simulink model "parallel_8_phase_voltages"  (R2022a)
settings: Solver=FixedStepDiscrete  StartTime=0.0  StopTime=10.0  RelTol=1e-3
undefined symbols (not defined in the file or in its folder): f_c, u_dc
libraries: hdlsllib x4, simulink x2
settings Model: DataTypeOverride=Off  Creator=Andre Merx  LastModifiedBy=Andre Merx
settings SolverCC: AlgebraicLoopSolver=TrustRegion
settings DataIOCC: LimitDataPoints=on  SaveOutput=off  SaveTime=off
settings OptimizationCC: BlockReduction=off  ConditionallyExecuteInputs=off  DefaultParameterBehavior=Inlined  LifeSpan=inf
settings DebuggingCC: AlgebraicLoopMsg=error  SingleTaskRateTransMsg=error  UnconnectedInputMsg=warning  UnconnectedOutputMsg=warning  UnconnectedLineMsg=warning  AllowSymbolicDim=off  StrictBusMsg=ErrorOnBusTreatedAsVector  SFUnexpectedBacktrackingDiag=warning  SFNoUnconditionalDefaultTransitionDiag=warning  SFExecutionAtInitializationDiag=none  SFMachineParentedDataDiag=warning  ArithmeticOperatorsInVariantConditions=warning
settings HardwareCC: ProdBitPerPointer=32  ProdBitPerSizeT=32  ProdBitPerPtrDiffT=32  ProdLargestAtomicFloat=None  ProdIntDivRoundTo=Undefined  ProdEndianess=Unspecified  ProdWordSize=32  ProdHWDeviceType=ASIC/FPGA->ASIC/FPGA  ProdEqTarget=off
settings SFSimCC: SimUseLocalCustomCode=off  CustomCodeUndefinedFunction=UseInterfaceOnly
settings RTWCC: RTWUseLocalCustomCode=off
settings CodeAppCC: StateflowObjectComments=on
settings GRTTargetCC: TargetLangStandard=C89/C90 (ANSI)
settings ConfigComp: CovScope=ReferencedModels  CovMetricSettings=dw  CovSaveCumulativeToWorkspaceVar=on  CovSaveSingleToWorkspaceVar=on  CovExternalEMLEnable=off  CovSFcnEnable=off

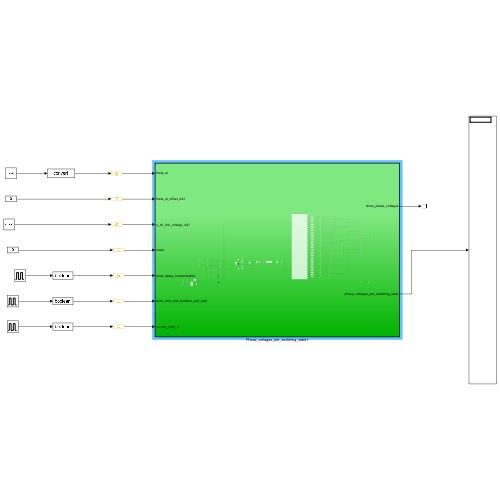
[thumbnail: Simulink's stored preview of the top-level diagram]
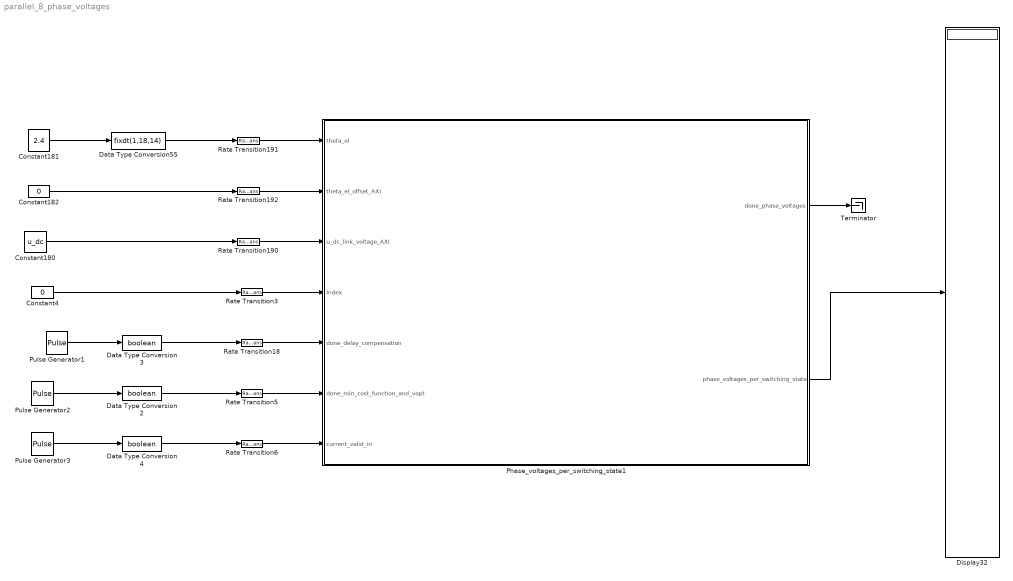
== system parallel_8_phase_voltages ==
  Constant180 : Constant  Value=u_dc  OutDataTypeStr=single  SampleTime=-1
  Constant181 : Constant  Value=2.4
  Constant182 : Constant  Value=0  OutDataTypeStr=fixdt(1,18,14)  SampleTime=-1
  Constant4 : Constant  Value=0  OutDataTypeStr=int32  SampleTime=-1
  Data Type Conversion2 : DataTypeConversion  OutDataTypeStr=boolean  SaturateOnIntegerOverflow=off  RndMeth=Floor
  Data Type Conversion3 : DataTypeConversion  OutDataTypeStr=boolean  SaturateOnIntegerOverflow=off  RndMeth=Floor
  Data Type Conversion4 : DataTypeConversion  OutDataTypeStr=boolean  SaturateOnIntegerOverflow=off  RndMeth=Floor
  Data Type Conversion55 : DataTypeConversion  OutDataTypeStr=fixdt(1,18,14)  SaturateOnIntegerOverflow=off  RndMeth=Floor
  Display32 : Display
  Phase_voltages_per_switching_state1 : Subsystem  TreatAsAtomicUnit=on
  Pulse Generator1 : DiscretePulseGenerator  PulseType=Time based  Period=1/f_c
  Pulse Generator2 : DiscretePulseGenerator  PulseType=Time based  Period=1/f_c
  Pulse Generator3 : DiscretePulseGenerator  PulseType=Time based  Period=1/f_c
  Rate Transition{3,5..6,18,190..192} (7 alike) : RateTransition  OutPortSampleTime=Rt
  Terminator : Terminator
  wires:
  Constant181/1 -> Data Type Conversion55/1
  Data Type Conversion55/1 -> Rate Transition191/1
  Constant180/1 -> Rate Transition190/1
  Constant182/1 -> Rate Transition192/1
  Rate Transition192/1 -> Phase_voltages_per_switching_state1/2(theta_el_offset_AXI)
  Phase_voltages_per_switching_state1/2(phase_voltages_per_switching_state) -> Display32/1
  Rate Transition191/1 -> Phase_voltages_per_switching_state1/1(theta_el)
  Rate Transition190/1 -> Phase_voltages_per_switching_state1/3(u_dc_link_voltage_AXI)
  Phase_voltages_per_switching_state1/1(done_phase_voltages) -> Terminator/1
  Pulse Generator2/1 -> Data Type Conversion2/1
  Rate Transition5/1 -> Phase_voltages_per_switching_state1/6(done_min_cost_function_and_vopt)
  Pulse Generator1/1 -> Data Type Conversion3/1
  Pulse Generator3/1 -> Data Type Conversion4/1
  Constant4/1 -> Rate Transition3/1
  Data Type Conversion4/1 -> Rate Transition6/1
  Data Type Conversion3/1 -> Rate Transition18/1
  Rate Transition18/1 -> Phase_voltages_per_switching_state1/5(done_delay_compensation)
  Rate Transition6/1 -> Phase_voltages_per_switching_state1/7(current_valid_in)
  Data Type Conversion2/1 -> Rate Transition5/1
  Rate Transition3/1 -> Phase_voltages_per_switching_state1/4(Index)

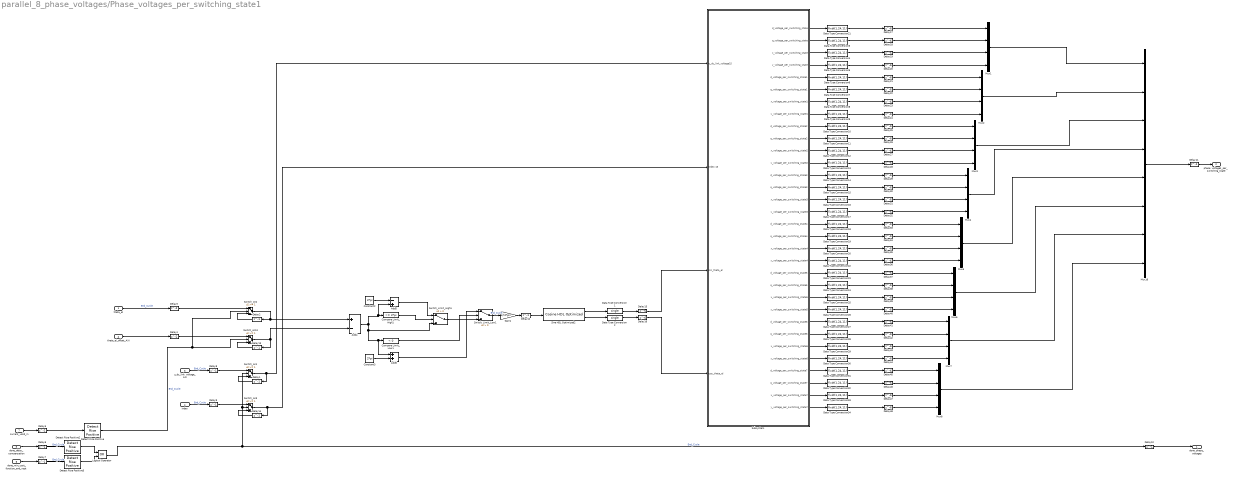
== system parallel_8_phase_voltages/Phase_voltages_per_switching_state1 ==
  theta_el : Inport
  theta_el_offset_AXI : Inport  Port=2
  u_dc_link_voltage_AXI : Inport  Port=3
  Index : Inport  Port=4
  done_delay_compensation : Inport  Port=5
  done_min_cost_function_and_vopt : Inport  Port=6
  current_valid_in : Inport  Port=7
  Add4 : Sum  Inputs=+-  OutDataTypeStr=Inherit: Same as first input
  Add5 : Sum  Inputs=-+  OutDataTypeStr=Inherit: Same as first input
  Add6 : Sum  OutDataTypeStr=Inherit: Same as first input
  Compare Limit_High1 : simulink/Logic and Bit Operations/Compare To Constant  relop=>=  const=2*pi  OutDataTypeStr=boolean
  Compare Limit_Low1 : simulink/Logic and Bit Operations/Compare To Constant  relop=<  const=0  OutDataTypeStr=boolean
  Constant2 : Constant  Value=2*pi  OutDataTypeStr=fixdt(1,18,14)  SampleTime=1/100000000
  Constant3 : Constant  Value=2*pi  OutDataTypeStr=fixdt(1,18,14)  SampleTime=1/100000000
  Data Type Conversion1 : DataTypeConversion  OutDataTypeStr=single  SaturateOnIntegerOverflow=off  RndMeth=Floor
  Data Type Conversion{3..34} (32 alike) : DataTypeConversion  OutDataTypeStr=fixdt(1,24,11)  SaturateOnIntegerOverflow=off  RndMeth=Floor
  Data Type Conversion2 : DataTypeConversion  OutDataTypeStr=single  SaturateOnIntegerOverflow=off  RndMeth=Floor
  Delay{1..2,6..14} (11 alike) : Delay  DelayLength=1
  Delay{15..48} (34 alike) : Delay  DelayLength=6
  Delay3 : Delay
  Delay4 : Delay
  Delay5 : Delay
  Detect Rise Positive : hdlsllib/Logic and Bit Operations/Detect Rise Positive  vinit=0  OutDataTypeStr=boolean
      settings: SourceProductBaseCode=SL
  Detect Rise Positive2 : hdlsllib/Logic and Bit Operations/Detect Rise Positive  vinit=0  OutDataTypeStr=boolean
      settings: SourceProductBaseCode=SL
  Detect Rise Positive3 : hdlsllib/Logic and Bit Operations/Detect Rise Positive  vinit=0  OutDataTypeStr=boolean
      settings: SourceProductBaseCode=SL
  Gain1 : Gain  Gain=1/(2*pi)  OutDataTypeStr=Inherit: Same as input  ParamDataTypeStr=Inherit: Same as input
  Logical Operator : Logic  Operator=OR  AllPortsSameDT=off  OutDataTypeStr=boolean
  Mux{1..8} (8 alike) : Mux
  Mux16 : Mux  Inputs=8
  Sine HDL Optimized2 : hdlsllib/Lookup Tables/Cosine HDL Optimized  OutputFormula=sin(2*pi*u) and cos(2*pi*u)  NumDataPoints=512  TableDataTypeStr=fixdt(1,15,14)  SimulateLUTROMDelay=off
      settings: SourceProductBaseCode=SL
  Subsystem : Subsystem
  Switch_Limit_High1 : Switch  Criteria=u2 > Threshold  SaturateOnIntegerOverflow=off  InputSameDT=off  OutDataTypeStr=Inherit: Same as first input
  Switch_Limit_Low1 : Switch  Criteria=u2 > Threshold  SaturateOnIntegerOverflow=off  InputSameDT=off  OutDataTypeStr=Inherit: Same as first input
  Switch_on1 : Switch  Threshold=1  OutDataTypeStr=single  RndMeth=Simplest  SaturateOnIntegerOverflow=off  InputSameDT=off
  Switch_on13 : Switch  Threshold=1  RndMeth=Simplest  SaturateOnIntegerOverflow=off  InputSameDT=off  OutDataTypeStr=Inherit: Same as first input
  Switch_on2 : Switch  Threshold=1  RndMeth=Simplest  SaturateOnIntegerOverflow=off  InputSameDT=off  OutDataTypeStr=Inherit: Same as first input
  Switch_on3 : Switch  Threshold=1  OutDataTypeStr=int32  RndMeth=Simplest  SaturateOnIntegerOverflow=off  InputSameDT=off
  done_phase_voltages : Outport
  phase_voltages_per_switching_state : Outport  Port=2
  wires:
  Delay14/1 -> Switch_on3/3
  Delay13/1 -> Switch_on13/3
  Switch_on13/1 -> Delay13/1, Add4/2
  u_dc_link_voltage_AXI/1 -> Delay8/1  "End_Cycle"
  Switch_on1/1 -> Subsystem/1(u_dc_link_voltage15), Delay1/1
  Logical Operator/1 -> Delay10/1, Switch_on3/2, Switch_on1/2  "End_Cycle"
  Delay1/1 -> Switch_on1/3
  Index/1 -> Delay9/1  "End_Cycle"
  Switch_on3/1 -> Delay14/1, Subsystem/2(Index 15)
  Mux1/1 -> Mux16/1
  Mux2/1 -> Mux16/2
  Mux3/1 -> Mux16/3
  Mux4/1 -> Mux16/4
  Mux5/1 -> Mux16/5
  Mux6/1 -> Mux16/6
  Mux7/1 -> Mux16/7
  Mux8/1 -> Mux16/8
  Mux16/1 -> Delay11/1
  current_valid_in/1 -> Delay5/1
  done_delay_compensation/1 -> Delay6/1
  done_min_cost_function_and_vopt/1 -> Delay7/1
  theta_el/1 -> Delay3/1  "End_Cycle"
  Add4/1 -> Switch_Limit_High1/3, Add6/1, Compare Limit_Low1/1, Add5/2, Compare Limit_High1/1
  Compare Limit_Low1/1 -> Switch_Limit_Low1/2
  Add5/1 -> Switch_Limit_High1/1
  theta_el_offset_AXI/1 -> Delay4/1
  Constant3/1 -> Add6/2
  Constant2/1 -> Add5/1
  Compare Limit_High1/1 -> Switch_Limit_High1/2
  Add6/1 -> Switch_Limit_Low1/1
  Switch_Limit_High1/1 -> Switch_Limit_Low1/3
  Delay2/1 -> Switch_on2/3
  Switch_on2/1 -> Add4/1, Delay2/1
  Detect Rise Positive/1 -> Switch_on2/2, Switch_on13/2  "End_Cycle"
  Delay3/1 -> Switch_on2/1
  Delay4/1 -> Switch_on13/1
  Delay5/1 -> Detect Rise Positive/1
  Delay6/1 -> Detect Rise Positive2/1
  Delay7/1 -> Detect Rise Positive3/1
  Delay8/1 -> Switch_on1/1
  Delay9/1 -> Switch_on3/1
  Delay10/1 -> done_phase_voltages/1
  Delay11/1 -> phase_voltages_per_switching_state/1
  Sine HDL Optimized2/2 -> Data Type Conversion2/1
  Subsystem/1(d_voltage_per_switching_state) -> Data Type Conversion21/1
  Subsystem/2(q_voltage_per_switching_state) -> Data Type Conversion3/1
  Subsystem/3(x_voltage_per_switching_state) -> Data Type Conversion4/1
  Subsystem/4(y_voltage_per_switching_state) -> Data Type Conversion5/1
  Subsystem/5(d_voltage_per_switching_state1) -> Data Type Conversion6/1
  Subsystem/6(q_voltage_per_switching_state1) -> Data Type Conversion7/1
  Subsystem/7(x_voltage_per_switching_state1) -> Data Type Conversion8/1
  Subsystem/8(y_voltage_per_switching_state1) -> Data Type Conversion9/1
  Subsystem/9(d_voltage_per_switching_state2) -> Data Type Conversion10/1
  Subsystem/10(q_voltage_per_switching_state2) -> Data Type Conversion11/1
  Subsystem/11(x_voltage_per_switching_state2) -> Data Type Conversion12/1
  Subsystem/12(y_voltage_per_switching_state2) -> Data Type Conversion13/1
  Subsystem/13(d_voltage_per_switching_state3) -> Data Type Conversion14/1
  Subsystem/14(q_voltage_per_switching_state3) -> Data Type Conversion15/1
  Subsystem/15(x_voltage_per_switching_state3) -> Data Type Conversion16/1
  Subsystem/16(y_voltage_per_switching_state3) -> Data Type Conversion17/1
  Subsystem/17(d_voltage_per_switching_state4) -> Data Type Conversion18/1
  Subsystem/18(q_voltage_per_switching_state4) -> Data Type Conversion19/1
  Subsystem/19(x_voltage_per_switching_state4) -> Data Type Conversion20/1
  Subsystem/20(y_voltage_per_switching_state4) -> Data Type Conversion22/1
  Subsystem/21(d_voltage_per_switching_state5) -> Data Type Conversion23/1
  Subsystem/22(q_voltage_per_switching_state5) -> Data Type Conversion24/1
  Subsystem/23(x_voltage_per_switching_state5) -> Data Type Conversion25/1
  Subsystem/24(y_voltage_per_switching_state5) -> Data Type Conversion26/1
  Subsystem/25(d_voltage_per_switching_state6) -> Data Type Conversion27/1
  Subsystem/26(q_voltage_per_switching_state6) -> Data Type Conversion28/1
  Subsystem/27(x_voltage_per_switching_state6) -> Data Type Conversion29/1
  Subsystem/28(y_voltage_per_switching_state6) -> Data Type Conversion30/1
  Subsystem/29(d_voltage_per_switching_state7) -> Data Type Conversion31/1
  Subsystem/30(q_voltage_per_switching_state7) -> Data Type Conversion32/1
  Subsystem/31(x_voltage_per_switching_state7) -> Data Type Conversion33/1
  Subsystem/32(y_voltage_per_switching_state7) -> Data Type Conversion34/1
  Sine HDL Optimized2/1 -> Data Type Conversion1/1
  Data Type Conversion2/1 -> Delay16/1
  Data Type Conversion1/1 -> Delay15/1
  Gain1/1 -> Delay12/1
  Delay12/1 -> Sine HDL Optimized2/1
  Switch_Limit_Low1/1 -> Gain1/1  "End_Cycle"
  Data Type Conversion21/1 -> Delay17/1
  Data Type Conversion3/1 -> Delay18/1
  Data Type Conversion4/1 -> Delay19/1
  Data Type Conversion5/1 -> Delay20/1
  Data Type Conversion6/1 -> Delay21/1
  Data Type Conversion7/1 -> Delay22/1
  Data Type Conversion8/1 -> Delay23/1
  Data Type Conversion9/1 -> Delay24/1
  Data Type Conversion10/1 -> Delay25/1
  Data Type Conversion11/1 -> Delay26/1
  Data Type Conversion12/1 -> Delay27/1
  Data Type Conversion13/1 -> Delay28/1
  Data Type Conversion14/1 -> Delay29/1
  Data Type Conversion15/1 -> Delay30/1
  Data Type Conversion16/1 -> Delay31/1
  Data Type Conversion17/1 -> Delay32/1
  Data Type Conversion18/1 -> Delay33/1
  Data Type Conversion19/1 -> Delay34/1
  Data Type Conversion20/1 -> Delay35/1
  Data Type Conversion22/1 -> Delay36/1
  Data Type Conversion23/1 -> Delay37/1
  Data Type Conversion24/1 -> Delay38/1
  Data Type Conversion25/1 -> Delay39/1
  Data Type Conversion26/1 -> Delay40/1
  Data Type Conversion27/1 -> Delay41/1
  Data Type Conversion28/1 -> Delay42/1
  Data Type Conversion29/1 -> Delay43/1
  Data Type Conversion30/1 -> Delay44/1
  Data Type Conversion31/1 -> Delay45/1
  Data Type Conversion32/1 -> Delay46/1
  Data Type Conversion33/1 -> Delay47/1
  Data Type Conversion34/1 -> Delay48/1
  Delay15/1 -> Subsystem/3(sin_theta_el)
  Delay16/1 -> Subsystem/4(cos_theta_el)
  Delay17/1 -> Mux1/1
  Delay18/1 -> Mux1/2
  Delay19/1 -> Mux1/3
  Delay20/1 -> Mux1/4
  Delay21/1 -> Mux2/1
  Delay22/1 -> Mux2/2
  Delay23/1 -> Mux2/3
  Delay24/1 -> Mux2/4
  Delay25/1 -> Mux3/1
  Delay26/1 -> Mux3/2
  Delay27/1 -> Mux3/3
  Delay28/1 -> Mux3/4
  Delay29/1 -> Mux4/1
  Delay30/1 -> Mux4/2
  Delay31/1 -> Mux4/3
  Delay32/1 -> Mux4/4
  Delay33/1 -> Mux5/1
  Delay34/1 -> Mux5/2
  Delay35/1 -> Mux5/3
  Delay36/1 -> Mux5/4
  Delay37/1 -> Mux6/1
  Delay38/1 -> Mux6/2
  Delay39/1 -> Mux6/3
  Delay40/1 -> Mux6/4
  Delay41/1 -> Mux7/1
  Delay42/1 -> Mux7/2
  Delay43/1 -> Mux7/3
  Delay44/1 -> Mux7/4
  Delay45/1 -> Mux8/1
  Delay46/1 -> Mux8/2
  Delay47/1 -> Mux8/3
  Delay48/1 -> Mux8/4
  Detect Rise Positive2/1 -> Logical Operator/1  "End_Cycle"
  Detect Rise Positive3/1 -> Logical Operator/2  "End_Cycle"

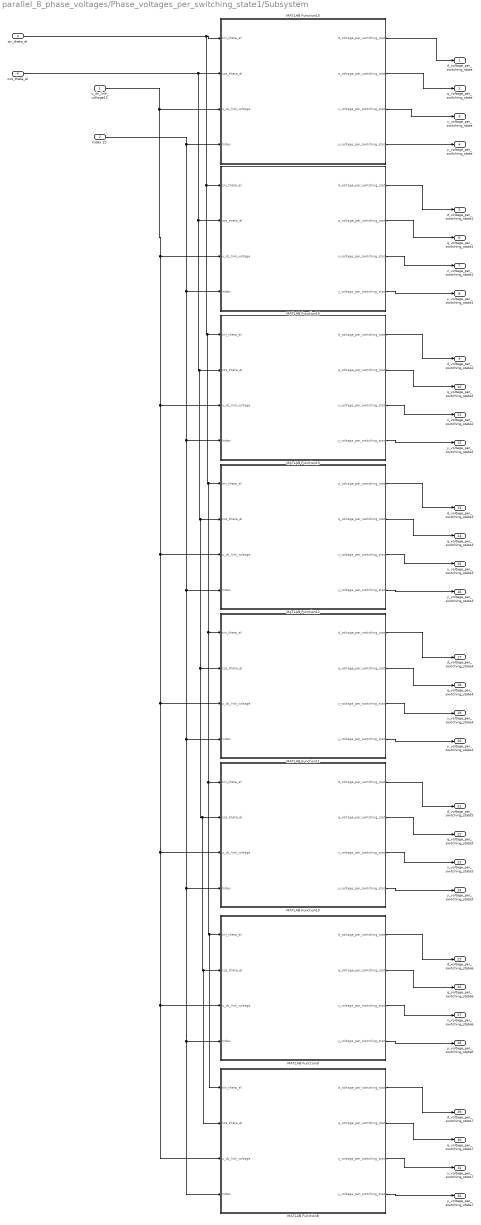
== system parallel_8_phase_voltages/Phase_voltages_per_switching_state1/Subsystem ==
  u_dc_link_voltage15 : Inport
  Index 15 : Inport  Port=2
  sin_theta_el : Inport  Port=3
  cos_theta_el : Inport  Port=4
  MATLAB Function10 : MATLAB Function  TreatAsAtomicUnit=on  SystemSampleTime=1/100000000
  MATLAB Function11 : MATLAB Function  TreatAsAtomicUnit=on  SystemSampleTime=1/100000000
  MATLAB Function12 : MATLAB Function  TreatAsAtomicUnit=on  SystemSampleTime=1/100000000
  MATLAB Function13 : MATLAB Function  TreatAsAtomicUnit=on  SystemSampleTime=1/100000000
  MATLAB Function14 : MATLAB Function  TreatAsAtomicUnit=on  SystemSampleTime=1/100000000
  MATLAB Function15 : MATLAB Function  TreatAsAtomicUnit=on  SystemSampleTime=1/100000000
  MATLAB Function8 : MATLAB Function  TreatAsAtomicUnit=on  SystemSampleTime=1/100000000
  MATLAB Function9 : MATLAB Function  TreatAsAtomicUnit=on  SystemSampleTime=1/100000000
  d_voltage_per_switching_state : Outport
  q_voltage_per_switching_state : Outport  Port=2
  x_voltage_per_switching_state : Outport  Port=3
  y_voltage_per_switching_state : Outport  Port=4
  d_voltage_per_switching_state1 : Outport  Port=5
  q_voltage_per_switching_state1 : Outport  Port=6
  x_voltage_per_switching_state1 : Outport  Port=7
  y_voltage_per_switching_state1 : Outport  Port=8
  d_voltage_per_switching_state2 : Outport  Port=9
  q_voltage_per_switching_state2 : Outport  Port=10
  x_voltage_per_switching_state2 : Outport  Port=11
  y_voltage_per_switching_state2 : Outport  Port=12
  d_voltage_per_switching_state3 : Outport  Port=13
  q_voltage_per_switching_state3 : Outport  Port=14
  x_voltage_per_switching_state3 : Outport  Port=15
  y_voltage_per_switching_state3 : Outport  Port=16
  d_voltage_per_switching_state4 : Outport  Port=17
  q_voltage_per_switching_state4 : Outport  Port=18
  x_voltage_per_switching_state4 : Outport  Port=19
  y_voltage_per_switching_state4 : Outport  Port=20
  d_voltage_per_switching_state5 : Outport  Port=21
  q_voltage_per_switching_state5 : Outport  Port=22
  x_voltage_per_switching_state5 : Outport  Port=23
  y_voltage_per_switching_state5 : Outport  Port=24
  d_voltage_per_switching_state6 : Outport  Port=25
  q_voltage_per_switching_state6 : Outport  Port=26
  x_voltage_per_switching_state6 : Outport  Port=27
  y_voltage_per_switching_state6 : Outport  Port=28
  d_voltage_per_switching_state7 : Outport  Port=29
  q_voltage_per_switching_state7 : Outport  Port=30
  x_voltage_per_switching_state7 : Outport  Port=31
  y_voltage_per_switching_state7 : Outport  Port=32
  wires:
  MATLAB Function11/4(y_voltage_per_switching_state) -> y_voltage_per_switching_state4/1
  MATLAB Function10/3(x_voltage_per_switching_state) -> x_voltage_per_switching_state5/1
  MATLAB Function8/1(d_voltage_per_switching_state) -> d_voltage_per_switching_state7/1
  MATLAB Function8/2(q_voltage_per_switching_state) -> q_voltage_per_switching_state7/1
  MATLAB Function11/1(d_voltage_per_switching_state) -> d_voltage_per_switching_state4/1
  MATLAB Function12/3(x_voltage_per_switching_state) -> x_voltage_per_switching_state3/1
  MATLAB Function15/2(q_voltage_per_switching_state) -> q_voltage_per_switching_state/1
  MATLAB Function8/3(x_voltage_per_switching_state) -> x_voltage_per_switching_state7/1
  MATLAB Function11/3(x_voltage_per_switching_state) -> x_voltage_per_switching_state4/1
  MATLAB Function10/4(y_voltage_per_switching_state) -> y_voltage_per_switching_state5/1
  MATLAB Function11/2(q_voltage_per_switching_state) -> q_voltage_per_switching_state4/1
  MATLAB Function12/1(d_voltage_per_switching_state) -> d_voltage_per_switching_state3/1
  MATLAB Function12/4(y_voltage_per_switching_state) -> y_voltage_per_switching_state3/1
  MATLAB Function13/2(q_voltage_per_switching_state) -> q_voltage_per_switching_state2/1
  MATLAB Function10/1(d_voltage_per_switching_state) -> d_voltage_per_switching_state5/1
  MATLAB Function10/2(q_voltage_per_switching_state) -> q_voltage_per_switching_state5/1
  MATLAB Function13/4(y_voltage_per_switching_state) -> y_voltage_per_switching_state2/1
  MATLAB Function8/4(y_voltage_per_switching_state) -> y_voltage_per_switching_state7/1
  MATLAB Function13/1(d_voltage_per_switching_state) -> d_voltage_per_switching_state2/1
  MATLAB Function13/3(x_voltage_per_switching_state) -> x_voltage_per_switching_state2/1
  MATLAB Function12/2(q_voltage_per_switching_state) -> q_voltage_per_switching_state3/1
  MATLAB Function15/1(d_voltage_per_switching_state) -> d_voltage_per_switching_state/1
  MATLAB Function15/4(y_voltage_per_switching_state) -> y_voltage_per_switching_state/1
  MATLAB Function15/3(x_voltage_per_switching_state) -> x_voltage_per_switching_state/1
  u_dc_link_voltage15/1 -> MATLAB Function8/3(u_dc_link_voltage), MATLAB Function9/3(u_dc_link_voltage), MATLAB Function10/3(u_dc_link_voltage), MATLAB Function11/3(u_dc_link_voltage), MATLAB Function12/3(u_dc_link_voltage), MATLAB Function13/3(u_dc_link_voltage), MATLAB Function14/3(u_dc_link_voltage), MATLAB Function15/3(u_dc_link_voltage)
  MATLAB Function14/4(y_voltage_per_switching_state) -> y_voltage_per_switching_state1/1
  MATLAB Function14/3(x_voltage_per_switching_state) -> x_voltage_per_switching_state1/1
  MATLAB Function14/1(d_voltage_per_switching_state) -> d_voltage_per_switching_state1/1
  MATLAB Function14/2(q_voltage_per_switching_state) -> q_voltage_per_switching_state1/1
  Index 15/1 -> MATLAB Function15/4(Index), MATLAB Function10/4(Index), MATLAB Function8/4(Index), MATLAB Function9/4(Index), MATLAB Function11/4(Index), MATLAB Function12/4(Index), MATLAB Function13/4(Index), MATLAB Function14/4(Index)
  MATLAB Function9/3(x_voltage_per_switching_state) -> x_voltage_per_switching_state6/1
  MATLAB Function9/2(q_voltage_per_switching_state) -> q_voltage_per_switching_state6/1
  MATLAB Function9/1(d_voltage_per_switching_state) -> d_voltage_per_switching_state6/1
  MATLAB Function9/4(y_voltage_per_switching_state) -> y_voltage_per_switching_state6/1
  sin_theta_el/1 -> MATLAB Function14/1(sin_theta_el), MATLAB Function8/1(sin_theta_el), MATLAB Function9/1(sin_theta_el), MATLAB Function10/1(sin_theta_el), MATLAB Function11/1(sin_theta_el), MATLAB Function12/1(sin_theta_el), MATLAB Function13/1(sin_theta_el), MATLAB Function15/1(sin_theta_el)
  cos_theta_el/1 -> MATLAB Function15/2(cos_theta_el), MATLAB Function8/2(cos_theta_el), MATLAB Function9/2(cos_theta_el), MATLAB Function10/2(cos_theta_el), MATLAB Function11/2(cos_theta_el), MATLAB Function12/2(cos_theta_el), MATLAB Function13/2(cos_theta_el), MATLAB Function14/2(cos_theta_el)

== matlab function parallel_8_phase_voltages/Phase_voltages_per_switching_state1/Subsystem/MATLAB Function9 ==
  data: sin_theta_el input; cos_theta_el input; d_voltage_per_switching_state output; u_dc_link_voltage input; Index input; q_voltage_per_switching_state output; x_voltage_per_switching_state output; y_voltage_per_switching_state output
function [d_voltage_per_switching_state, q_voltage_per_switching_state, x_voltage_per_switching_state, y_voltage_per_switching_state] = fcn(sin_theta_el, cos_theta_el, u_dc_link_voltage, Index)
      
        % Initial condition
            Index = Index+1;

    
        % Swichtingstates factors alpha beta x y
        Factors_alpha_beta_x_y = single([-0.288675134594813	 0.0446581987385205  -0.455341801261480	  -0.122008467928146    -0.455341801261480	-0.122008467928146	-0.622008467928146	-0.288675134594813;
                                         -0.166666666666667	-0.166666666666667	  0.122008467928146	   0.122008467928146    -0.455341801261480	-0.455341801261480	-0.166666666666667	-0.166666666666667;
                                         0.288675134594813	 0.622008467928146	  0.122008467928146	   0.455341801261480     0.122008467928146	 0.455341801261480	-0.0446581987385205  0.288675134594813;
                                         -0.166666666666667	-0.166666666666667	 -0.455341801261480	  -0.455341801261480     0.122008467928146	 0.122008467928146	-0.166666666666667	-0.166666666666667]);
        
        % Park-Transformation of the switchingstates factors
        Factors_d_q_x_y =single(zeros(4,1));
    
        Factors_d_q_x_y(3,1) = Factors_alpha_beta_x_y(3,Index);
        Factors_d_q_x_y(4,1) = Factors_alpha_beta_x_y(4,Index);
       
        Factors_d_q_x_y(1,1) = cos_theta_el*Factors_alpha_beta_x_y(1,Index)+sin_theta_el*Factors_alpha_beta_x_y(2,Index);
        Factors_d_q_x_y(2,1) = -sin_theta_el*Factors_alpha_beta_x_y(1,Index)+cos_theta_el*Factors_alpha_beta_x_y(2,Index);
    
        %Calculation of the voltages per switching state in alpha beta coordinates
        d_q_x_y_voltages_per_switching_state = single(u_dc_link_voltage*Factors_d_q_x_y);
    
        d_voltage_per_switching_state = d_q_x_y_voltages_per_switching_state(1,1);
        q_voltage_per_switching_state = d_q_x_y_voltages_per_switching_state(2,1);
        x_voltage_per_switching_state = d_q_x_y_voltages_per_switching_state(3,1);
        y_voltage_per_switching_state = d_q_x_y_voltages_per_switching_state(4,1);
    

end

== matlab function parallel_8_phase_voltages/Phase_voltages_per_switching_state1/Subsystem/MATLAB Function10 ==
  data: sin_theta_el input; cos_theta_el input; d_voltage_per_switching_state output; u_dc_link_voltage input; Index input; q_voltage_per_switching_state output; x_voltage_per_switching_state output; y_voltage_per_switching_state output
function [d_voltage_per_switching_state, q_voltage_per_switching_state, x_voltage_per_switching_state, y_voltage_per_switching_state] = fcn(sin_theta_el, cos_theta_el, u_dc_link_voltage, Index)
      
        % Initial condition
            Index = Index+1;

        % Swichtingstates factors alpha beta x y
        Factors_alpha_beta_x_y = single([0.288675134594813	 0.622008467928146	 0.122008467928146	 0.455341801261480    0.122008467928146	 0.455341801261480	-0.0446581987385205  0.288675134594813;
                                         -0.166666666666667	-0.166666666666667	 0.122008467928146	 0.122008467928146   -0.455341801261480	-0.455341801261480	-0.166666666666667	-0.166666666666667;
                                         -0.288675134594813	 0.0446581987385205	-0.455341801261480	-0.122008467928146   -0.455341801261480	-0.122008467928146	-0.622008467928146	-0.288675134594813;
                                         -0.166666666666667	-0.166666666666667	-0.455341801261480	-0.455341801261480    0.122008467928146	 0.122008467928146	-0.166666666666667	-0.166666666666667]);
        
        % Park-Transformation of the switchingstates factors
        Factors_d_q_x_y =single(zeros(4,1));
    
        Factors_d_q_x_y(3,1) = Factors_alpha_beta_x_y(3,Index);
        Factors_d_q_x_y(4,1) = Factors_alpha_beta_x_y(4,Index);
       
        Factors_d_q_x_y(1,1) = cos_theta_el*Factors_alpha_beta_x_y(1,Index)+sin_theta_el*Factors_alpha_beta_x_y(2,Index);
        Factors_d_q_x_y(2,1) = -sin_theta_el*Factors_alpha_beta_x_y(1,Index)+cos_theta_el*Factors_alpha_beta_x_y(2,Index);
    
        %Calculation of the voltages per switching state in alpha beta coordinates
        d_q_x_y_voltages_per_switching_state = single(u_dc_link_voltage*Factors_d_q_x_y);
    
        d_voltage_per_switching_state = d_q_x_y_voltages_per_switching_state(1,1);
        q_voltage_per_switching_state = d_q_x_y_voltages_per_switching_state(2,1);
        x_voltage_per_switching_state = d_q_x_y_voltages_per_switching_state(3,1);
        y_voltage_per_switching_state = d_q_x_y_voltages_per_switching_state(4,1);
    

end

== matlab function parallel_8_phase_voltages/Phase_voltages_per_switching_state1/Subsystem/MATLAB Function11 ==
  data: sin_theta_el input; cos_theta_el input; d_voltage_per_switching_state output; u_dc_link_voltage input; Index input; q_voltage_per_switching_state output; x_voltage_per_switching_state output; y_voltage_per_switching_state output
function [d_voltage_per_switching_state, q_voltage_per_switching_state, x_voltage_per_switching_state, y_voltage_per_switching_state] = fcn(sin_theta_el, cos_theta_el, u_dc_link_voltage, Index)
      
        % Initial condition
            Index = Index+1;

    
        % Swichtingstates factors alpha beta x y
        Factors_alpha_beta_x_y = single([0	                 0.333333333333333	-0.166666666666667	  0.166666666666667    -0.166666666666667	  0.166666666666667	    -0.333333333333333	 0;
                                        -0.333333333333333	-0.333333333333333	-0.0446581987385205	 -0.0446581987385205   -0.622008467928146	 -0.622008467928146	    -0.333333333333333	-0.333333333333333;
                                         0	                 0.333333333333333	-0.166666666666667	  0.166666666666667    -0.166666666666667	  0.166666666666667	    -0.333333333333333	 0;
                                        -0.333333333333333	-0.333333333333333	-0.622008467928146	 -0.622008467928146    -0.0446581987385205   -0.0446581987385205	-0.333333333333333	-0.333333333333333]);
        
        % Park-Transformation of the switchingstates factors
        Factors_d_q_x_y =single(zeros(4,1));
    
        Factors_d_q_x_y(3,1) = Factors_alpha_beta_x_y(3,Index);
        Factors_d_q_x_y(4,1) = Factors_alpha_beta_x_y(4,Index);

        Factors_d_q_x_y(1,1) = cos_theta_el*Factors_alpha_beta_x_y(1,Index)+sin_theta_el*Factors_alpha_beta_x_y(2,Index);
        Factors_d_q_x_y(2,1) = -sin_theta_el*Factors_alpha_beta_x_y(1,Index)+cos_theta_el*Factors_alpha_beta_x_y(2,Index);
    
        %Calculation of the voltages per switching state in alpha beta coordinates
        d_q_x_y_voltages_per_switching_state = single(u_dc_link_voltage*Factors_d_q_x_y);
    
        d_voltage_per_switching_state = d_q_x_y_voltages_per_switching_state(1,1);
        q_voltage_per_switching_state = d_q_x_y_voltages_per_switching_state(2,1);
        x_voltage_per_switching_state = d_q_x_y_voltages_per_switching_state(3,1);
        y_voltage_per_switching_state = d_q_x_y_voltages_per_switching_state(4,1);
    

end

== matlab function parallel_8_phase_voltages/Phase_voltages_per_switching_state1/Subsystem/MATLAB Function12 ==
  data: sin_theta_el input; cos_theta_el input; d_voltage_per_switching_state output; u_dc_link_voltage input; Index input; q_voltage_per_switching_state output; x_voltage_per_switching_state output; y_voltage_per_switching_state output
function [d_voltage_per_switching_state, q_voltage_per_switching_state, x_voltage_per_switching_state, y_voltage_per_switching_state] = fcn(sin_theta_el, cos_theta_el, u_dc_link_voltage, Index)
      
        % Initial condition
            Index = Index+1;

    
        % Swichtingstates factors alpha beta x y
        Factors_alpha_beta_x_y = single([0	                0.333333333333333	-0.166666666666667  	0.166666666666667   -0.166666666666667	 0.166666666666667	 -0.333333333333333	0;
                                         0.333333333333333	0.333333333333333	 0.622008467928146	    0.622008467928146    0.0446581987385205	 0.0446581987385205	  0.333333333333333	0.333333333333333;
                                         0	                0.333333333333333	-0.166666666666667	    0.166666666666667   -0.166666666666667	 0.166666666666667	 -0.333333333333333	0;
                                         0.333333333333333	0.333333333333333	 0.0446581987385205 	0.0446581987385205   0.622008467928146	 0.622008467928146	  0.333333333333333	0.333333333333333]);
        
        % Park-Transformation of the switchingstates factors
        Factors_d_q_x_y =single(zeros(4,1));
    
        Factors_d_q_x_y(3,1) = Factors_alpha_beta_x_y(3,Index);
        Factors_d_q_x_y(4,1) = Factors_alpha_beta_x_y(4,Index);
           
        Factors_d_q_x_y(1,1) = cos_theta_el*Factors_alpha_beta_x_y(1,Index)+sin_theta_el*Factors_alpha_beta_x_y(2,Index);
        Factors_d_q_x_y(2,1) = -sin_theta_el*Factors_alpha_beta_x_y(1,Index)+cos_theta_el*Factors_alpha_beta_x_y(2,Index);
    
        %Calculation of the voltages per switching state in alpha beta coordinates
        d_q_x_y_voltages_per_switching_state = single(u_dc_link_voltage*Factors_d_q_x_y);
    
        d_voltage_per_switching_state = d_q_x_y_voltages_per_switching_state(1,1);
        q_voltage_per_switching_state = d_q_x_y_voltages_per_switching_state(2,1);
        x_voltage_per_switching_state = d_q_x_y_voltages_per_switching_state(3,1);
        y_voltage_per_switching_state = d_q_x_y_voltages_per_switching_state(4,1);
    

end

== matlab function parallel_8_phase_voltages/Phase_voltages_per_switching_state1/Subsystem/MATLAB Function13 ==
  data: sin_theta_el input; cos_theta_el input; d_voltage_per_switching_state output; u_dc_link_voltage input; Index input; q_voltage_per_switching_state output; x_voltage_per_switching_state output; y_voltage_per_switching_state output
function [d_voltage_per_switching_state, q_voltage_per_switching_state, x_voltage_per_switching_state, y_voltage_per_switching_state] = fcn(sin_theta_el, cos_theta_el, u_dc_link_voltage, Index)
      
        % Initial condition
            Index = Index+1;

    
        % Swichtingstates factors alpha beta x y
        Factors_alpha_beta_x_y = single([-0.288675134594813	0.0446581987385205	-0.455341801261480	-0.122008467928146   -0.455341801261480	-0.122008467928146	-0.622008467928146	-0.288675134594813;
                                         0.166666666666667	0.166666666666667	 0.455341801261480   0.455341801261480   -0.122008467928146	-0.122008467928146	 0.166666666666667	 0.166666666666667;
                                         0.288675134594813	0.622008467928146	 0.122008467928146	 0.455341801261480    0.122008467928146	 0.455341801261480	-0.0446581987385205	 0.288675134594813;
                                         0.166666666666667	0.166666666666667	-0.122008467928146	-0.122008467928146    0.455341801261480	 0.455341801261480	 0.166666666666667	 0.166666666666667]);
        
        % Park-Transformation of the switchingstates factors
        Factors_d_q_x_y =single(zeros(4,1));
    
        Factors_d_q_x_y(3,1) = Factors_alpha_beta_x_y(3,Index);
        Factors_d_q_x_y(4,1) = Factors_alpha_beta_x_y(4,Index);
           
        Factors_d_q_x_y(1,1) = cos_theta_el*Factors_alpha_beta_x_y(1,Index)+sin_theta_el*Factors_alpha_beta_x_y(2,Index);
        Factors_d_q_x_y(2,1) = -sin_theta_el*Factors_alpha_beta_x_y(1,Index)+cos_theta_el*Factors_alpha_beta_x_y(2,Index);
    
        %Calculation of the voltages per switching state in alpha beta coordinates
        d_q_x_y_voltages_per_switching_state = single(u_dc_link_voltage*Factors_d_q_x_y);
    
        d_voltage_per_switching_state = d_q_x_y_voltages_per_switching_state(1,1);
        q_voltage_per_switching_state = d_q_x_y_voltages_per_switching_state(2,1);
        x_voltage_per_switching_state = d_q_x_y_voltages_per_switching_state(3,1);
        y_voltage_per_switching_state = d_q_x_y_voltages_per_switching_state(4,1);
    

end

== matlab function parallel_8_phase_voltages/Phase_voltages_per_switching_state1/Subsystem/MATLAB Function14 ==
  data: sin_theta_el input; cos_theta_el input; d_voltage_per_switching_state output; u_dc_link_voltage input; Index input; q_voltage_per_switching_state output; x_voltage_per_switching_state output; y_voltage_per_switching_state output
function [d_voltage_per_switching_state, q_voltage_per_switching_state, x_voltage_per_switching_state, y_voltage_per_switching_state] = fcn(sin_theta_el, cos_theta_el, u_dc_link_voltage, Index)
      
        % Initial condition
            Index = Index+1;

    
        % Swichtingstates factors alpha beta x y
        Factors_alpha_beta_x_y = single([0.288675134594813	0.622008467928146	 0.122008467928146  	0.455341801261480     0.122008467928146	 0.455341801261480	-0.0446581987385205  0.288675134594813;   
                                         0.166666666666667	0.166666666666667	 0.455341801261480  	0.455341801261480    -0.122008467928146	-0.122008467928146	 0.166666666666667	 0.166666666666667;
                                         -0.288675134594813	0.0446581987385205	-0.455341801261480	   -0.122008467928146    -0.455341801261480	-0.122008467928146	-0.622008467928146	-0.288675134594813;
                                         0.166666666666667	0.166666666666667	-0.122008467928146     -0.122008467928146     0.455341801261480	 0.455341801261480	 0.166666666666667	 0.166666666666667]);
        
        % Park-Transformation of the switchingstates factors
        Factors_d_q_x_y =single(zeros(4,1));
    
        Factors_d_q_x_y(3,1) = Factors_alpha_beta_x_y(3,Index);
        Factors_d_q_x_y(4,1) = Factors_alpha_beta_x_y(4,Index);
       
        Factors_d_q_x_y(1,1) = cos_theta_el*Factors_alpha_beta_x_y(1,Index)+sin_theta_el*Factors_alpha_beta_x_y(2,Index);
        Factors_d_q_x_y(2,1) = -sin_theta_el*Factors_alpha_beta_x_y(1,Index)+cos_theta_el*Factors_alpha_beta_x_y(2,Index);
    
        %Calculation of the voltages per switching state in alpha beta coordinates
        d_q_x_y_voltages_per_switching_state = single(u_dc_link_voltage*Factors_d_q_x_y);
    
        d_voltage_per_switching_state = d_q_x_y_voltages_per_switching_state(1,1);
        q_voltage_per_switching_state = d_q_x_y_voltages_per_switching_state(2,1);
        x_voltage_per_switching_state = d_q_x_y_voltages_per_switching_state(3,1);
        y_voltage_per_switching_state = d_q_x_y_voltages_per_switching_state(4,1);
    

end

== matlab function parallel_8_phase_voltages/Phase_voltages_per_switching_state1/Subsystem/MATLAB Function15 ==
  data: sin_theta_el input; cos_theta_el input; d_voltage_per_switching_state output; u_dc_link_voltage input; Index input; q_voltage_per_switching_state output; x_voltage_per_switching_state output; y_voltage_per_switching_state output
function [d_voltage_per_switching_state, q_voltage_per_switching_state, x_voltage_per_switching_state, y_voltage_per_switching_state] = fcn(sin_theta_el, cos_theta_el, u_dc_link_voltage, Index)
      
        % Initial condition
            Index = Index+1;

        % Swichtingstates factors alpha beta x y
        Factors_alpha_beta_x_y = single([0	    0.333333333333333	-0.166666666666667	 0.166666666666667    -0.166666666666667	 0.166666666666667	-0.333333333333333	0;
                                         0	    0                    0.288675134594813	 0.288675134594813    -0.288675134594813	-0.288675134594813	 0	                0;
                                         0	    0.333333333333333	-0.166666666666667	 0.166666666666667    -0.166666666666667	 0.166666666666667	-0.333333333333333	0;
                                         0	    0	                -0.288675134594813	-0.288675134594813     0.288675134594813	 0.288675134594813	 0              	0]);
        
        % Park-Transformation of the switchingstates factors
        Factors_d_q_x_y =single(zeros(4,1));
    
        Factors_d_q_x_y(3,1) = Factors_alpha_beta_x_y(3,Index);
        Factors_d_q_x_y(4,1) = Factors_alpha_beta_x_y(4,Index);
          
        Factors_d_q_x_y(1,1) = cos_theta_el*Factors_alpha_beta_x_y(1,Index)+sin_theta_el*Factors_alpha_beta_x_y(2,Index);
        Factors_d_q_x_y(2,1) = -sin_theta_el*Factors_alpha_beta_x_y(1,Index)+cos_theta_el*Factors_alpha_beta_x_y(2,Index);
    
        %Calculation of the voltages per switching state in alpha beta coordinates
        d_q_x_y_voltages_per_switching_state = single(u_dc_link_voltage*Factors_d_q_x_y);
    
        d_voltage_per_switching_state = d_q_x_y_voltages_per_switching_state(1,1);
        q_voltage_per_switching_state = d_q_x_y_voltages_per_switching_state(2,1);
        x_voltage_per_switching_state = d_q_x_y_voltages_per_switching_state(3,1);
        y_voltage_per_switching_state = d_q_x_y_voltages_per_switching_state(4,1);
    

end

== matlab function parallel_8_phase_voltages/Phase_voltages_per_switching_state1/Subsystem/MATLAB Function8 ==
  data: sin_theta_el input; cos_theta_el input; d_voltage_per_switching_state output; u_dc_link_voltage input; Index input; q_voltage_per_switching_state output; x_voltage_per_switching_state output; y_voltage_per_switching_state output
function [d_voltage_per_switching_state, q_voltage_per_switching_state, x_voltage_per_switching_state, y_voltage_per_switching_state] = fcn(sin_theta_el, cos_theta_el, u_dc_link_voltage, Index)
      
        % Initial condition
            Index = Index+1;

    
        % Swichtingstates factors alpha beta x y
        Factors_alpha_beta_x_y = single([0	0.333333333333333	-0.166666666666667	 0.166666666666667    -0.166666666666667	 0.166666666666667	-0.333333333333333	0;
                                         0	0	                 0.288675134594813	 0.288675134594813    -0.288675134594813	-0.288675134594813	 0	                0;
                                         0	0.333333333333333	-0.166666666666667	 0.166666666666667    -0.166666666666667	 0.166666666666667	-0.333333333333333	0;
                                         0	0	                -0.288675134594813	-0.288675134594813     0.288675134594813	 0.288675134594813	 0	                0]);
        
        % Park-Transformation of the switchingstates factors
        Factors_d_q_x_y =single(zeros(4,1));
    
        Factors_d_q_x_y(3,1) = Factors_alpha_beta_x_y(3,Index);
        Factors_d_q_x_y(4,1) = Factors_alpha_beta_x_y(4,Index);
       
        Factors_d_q_x_y(1,1) = cos_theta_el*Factors_alpha_beta_x_y(1,Index)+sin_theta_el*Factors_alpha_beta_x_y(2,Index);
        Factors_d_q_x_y(2,1) = -sin_theta_el*Factors_alpha_beta_x_y(1,Index)+cos_theta_el*Factors_alpha_beta_x_y(2,Index);
    
        %Calculation of the voltages per switching state in alpha beta coordinates
        d_q_x_y_voltages_per_switching_state = single(u_dc_link_voltage*Factors_d_q_x_y);
    
        d_voltage_per_switching_state = d_q_x_y_voltages_per_switching_state(1,1);
        q_voltage_per_switching_state = d_q_x_y_voltages_per_switching_state(2,1);
        x_voltage_per_switching_state = d_q_x_y_voltages_per_switching_state(3,1);
        y_voltage_per_switching_state = d_q_x_y_voltages_per_switching_state(4,1);
    

end
